simulink model "TCT_and_SUDOKU"  (R2025a)
settings: Solver=VariableStepAuto  StartTime=0.0  StopTime=1  RelTol=1e-3
libraries: spsDiodeLib x162, spsPVArrayLib x162, spsControlledVoltageSourceLib x2, spsCurrentMeasurementLib x2, simulink x2, spsVoltageMeasurementLib x2, sps_lib x1
(part 1 of 2)
settings Model: Creator=waquarahmad  LastModifiedBy=waquarahmad

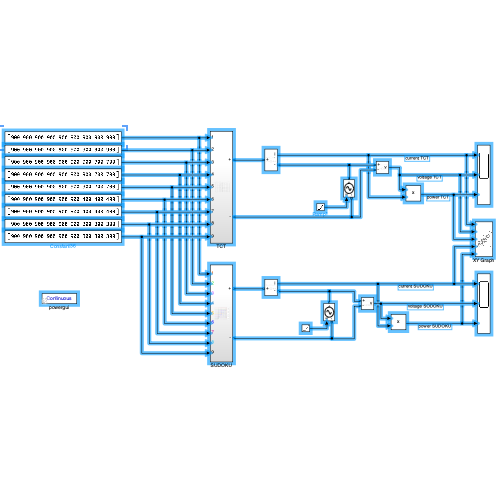
[thumbnail: Simulink's stored preview of the top-level diagram]
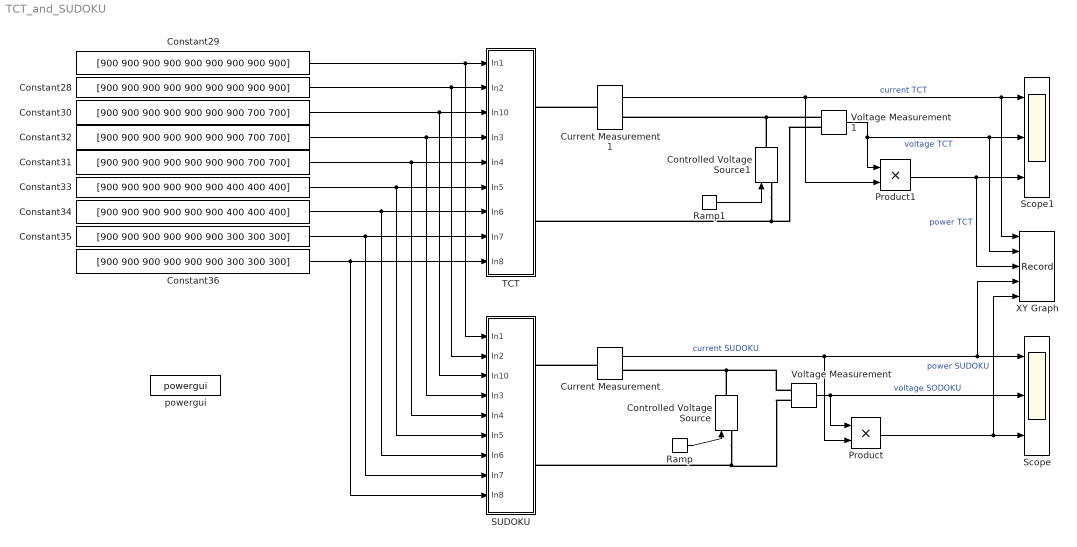
== system TCT_and_SUDOKU ==
  Constant28 : Constant  Value=[900 900 900 900 900 900 900 900 900]
  Constant29 : Constant  Value=[900 900 900 900 900 900 900 900 900]
  Constant30 : Constant  Value=[900 900 900 900 900 900 900 700 700]
  Constant31 : Constant  Value=[900 900 900 900 900 900 900 700 700]
  Constant32 : Constant  Value=[900 900 900 900 900 900 900 700 700]
  Constant33 : Constant  Value=[900 900 900 900 900 900 400 400 400]
  Constant34 : Constant  Value=[900 900 900 900 900 900 400 400 400]
  Constant35 : Constant  Value=[900 900 900 900 900 900 300 300 300]
  Constant36 : Constant  Value=[900 900 900 900 900 900 300 300 300]
  Controlled Voltage Source : spsControlledVoltageSourceLib/Controlled Voltage Source  Initialize=on  Source_Type=AC  Amplitude=0  Phase=0  Frequency=0  Measurements=None
  Controlled Voltage Source1 : spsControlledVoltageSourceLib/Controlled Voltage Source  Initialize=on  Source_Type=AC  Amplitude=0  Phase=0  Frequency=0  Measurements=None
  Current Measurement : spsCurrentMeasurementLib/Current Measurement  PhasorSimulation=off  OutputType=Complex  PSBequivalent=0
  Current Measurement1 : spsCurrentMeasurementLib/Current Measurement  PhasorSimulation=off  OutputType=Complex  PSBequivalent=0
  Product : Product
  Product1 : Product
  Ramp : simulink/Sources/Ramp  slope=22*9  start=0  InitialOutput=0
  Ramp1 : simulink/Sources/Ramp  slope=22*9  start=0  InitialOutput=0
  SUDOKU : Subsystem
  Scope : Scope  NumInputPorts=3
      settings: ActiveDisplayYMinimum=-11.703677982280553  ActiveDisplayYMaximum=43.6686902201964
  Scope1 : Scope  NumInputPorts=3
      settings: ActiveDisplayYMinimum=-1001.3880927326314  ActiveDisplayYMaximum=153.76114872783529
  TCT : Subsystem
  Voltage Measurement : spsVoltageMeasurementLib/Voltage Measurement  PhasorSimulation=off  OutputType=Complex  PSBequivalent=0
  Voltage Measurement1 : spsVoltageMeasurementLib/Voltage Measurement  PhasorSimulation=off  OutputType=Complex  PSBequivalent=0
  XY Graph : Record  NumPorts=5.0  FileSettingsInternal="{\"entries\":[{\"content\":{\"excelSettings\":{\"content\":{},\"type\":\"Streamout.ExcelSettings\"},\"parquetSettings\":{\"content\":{},\"type\":\"Streamout.ParquetSettings\"}},\"type\":\"Streamout.FileSettingStorage\",\"uuid\":\"\"}],\"packageUris\":[\"http:\\/\\/schema.mathworks.com\\/mf0\\/streamout_blocks\\/R2020a\"],\"version\":\"1.0\"}"  FrameSettings=[0, 0, 0, 0, 0]  Layout=[2 2]  SignalsInternal="{\"entries\":[{\"content\":{\"signals\":[{\"content\":{\"blockPath\":[],\"dimensions\":[1],\"domain\":\"\",\"lineColor\":\"#edb120\",\"lineWidth\":2,\"plots\":[ 2 ],\"port\":1,\"sid\":[\"\"],\"signalID\":1,\"signalName\":\"current TCT\"},\"type\":\"RecordBlkView.Signal\",\"uuid\":\"\"},{\"content\":{\"blockPath\":[],\"dimensions\":[1],\"domain\":\"\",\"lineColor\":\"#ff13a6\",\"lineWidth\":2,\"plots\":[ 1, 2 ],\"port\":2,\"sid\":[\"\"],\"signalID\":2,\"signalName\":\"voltage TCT\"},\"type\":\"RecordBlkView.Signal\",\"uuid\":\"\"},{\"content\":{\"blockPath\":[],\"dimensions\":[1],\"domain\":\"\",\"lineColor\":\"#fe330a\",\"lineWidth\":2,\"plots\":[ 1, 9 ],\"port\":3,\"sid\":[\"\"],\"signalID\":3,\"signalName\":\"power TCT\"},\"type\":\"RecordBlkView.Signal\",\"uuid\":\"\"},{\"content\":{\"blockPath\":[],\"dimensions\":[1],\"domain\":\"\",\"lineColor\":\"#22b573\",\"lineWidth\":2,\"plots\":[ 2 ],\"port\":4,\"sid\":[\"\"],\"signalID\":4,\"signalName\":\"current SUDOKU\"},\"type\":\"RecordBlkView.Signal\",\"uuid\":\"\"},{\"content\":{\"blockPath\":[],\"dimensions\":[1],\"domain\":\"\",\"lineColor\":\"#0072bd\",\"lineWidth\":2,\"plots\":[ 1, 10 ],\"port\":5,\"sid\":[\"\"],\"signalID\":5,\"signalName\":\"power SUDOKU\"},\"type\":\"RecordBlkView.Signal\",\"uuid\":\"\"}]},\"type\":\"RecordBlkView.InputSignals\",\"uuid\":\"\"}],\"packageUris\":[\"http:\\/\\/schema.mathworks.com\\/mf0\\/streamout_blocks\\/R2020a\"],\"version\":\"1.0\"}"  VisualizationBindings="{\"xyplotplugin\":{\"info\":[{\"series\":[{\"bindingParametersList\":[{\"parameter\":\"X-Axis\",\"signalID\":2,\"signalName\":\"voltage TCT\"},{\"parameter\":\"Y-Axis\",\"signalID\":5,\"signalName\":\"power SUDOKU\"},{\"parameter\":\"X-Axis\",\"signalID\":2,\"signalName\":\"voltage TCT\"},{\"parameter\":\"Y-Axis\",\"signalID\":5,\"signalName\":\"power SUDOKU\"}],\"seriesID\":0},{\"bindingParametersList\":[{\"parameter\":\"X-Axis\",\"signalID\":2,\"signalName\":\"voltage TCT\"},{\"parameter\":\"Y-Axis\",\"signalID\":3,\"signalName\":\"power TCT\"},{\"parameter\":\"X-Axis\",\"signalID\":2,\"signalName\":\"voltage TCT\"},{\"parameter\":\"Y-Axis\",\"signalID\":3,\"signalName\":\"power TCT\"}],\"seriesID\":1}],\"subplotID\":1},{\"series\":[{\"bindingParametersList\":[{\"parameter\":\"X-Axis\",\"signalID\":2,\"signalName\":\"voltage TCT\"},{\"parameter\":\"Y-Axis\",\"signalID\":1,\"signalName\":\"current TCT\"}],\"seriesID\":2},{\"bindingParametersList\":[{\"parameter\":\"X-Axis\",\"signalID\":2,\"signalName\":\"voltage TCT\"},{\"parameter\":\"Y-Axis\",\"signalID\":4,\"signalName\":\"current SUDOKU\"}],\"seriesID\":3}],\"subplotID\":2}]}}"  CompatibilityTag=XY
  powergui : sps_lib/powergui  Priority=1  SimulationMode=Continuous  SampleTime=1e-5  frequency=60  Iterations=50  frequencyindice=0  Pbase=100e6  ErrMax=1e-4  UnitsV=kV  UnitsW=MW  buscounter=0  FunctionMessages=off  echomessages=off  EnableUseOfTLC=off  CurrentSourceSwitches=off  DisableSnubberDevices=off  DisableRonSwitches=off  DisableVfSwitches=off  DisplayEquations=off  AutomaticDiscreteSolvers=off  SolverType=Tustin/Backward Euler (TBE)  Interpol=off  ExternalGateDelay=off  methode=off  Ts=100  x0status=blocks  SPID=on  SwTol=0  HookPort=off  NonlinearTolerance=1e-4  nMaxIteration=100  ContinueOnMaxIteration=off  RestoreLinks=warning  ResistiveCurrentMeasurement=off  Frange=[0:2:500]  Ylog=off  Xlog=on  ShowGrid=off  save=off  variable=ZData  structure=0  ZoomFFT=off  StartTime=0.0  cycles=1  DisplayStyle=1  fundamental=60  FreqAxis=off  MaxFrequency=1000  frequencyindicesteady=1  RmsSteady=1  display=off
  wires:
  Product/1 -> XY Graph/5, Scope/3  "power SUDOKU"
  Ramp/1 -> Controlled Voltage Source/1
  Voltage Measurement/1 -> Product/1, Scope/2  "voltage SODOKU"
  Current Measurement/1 -> Scope/1, XY Graph/4, Product/2  "current SUDOKU"
  Constant34/1 -> SUDOKU/7(In6), TCT/7(In6)
  Constant32/1 -> SUDOKU/4(In3), TCT/4(In3)
  Constant36/1 -> SUDOKU/9(In8), TCT/9(In8)
  Constant28/1 -> SUDOKU/2(In2), TCT/2(In2)
  Constant35/1 -> SUDOKU/8(In7), TCT/8(In7)
  Ramp1/1 -> Controlled Voltage Source1/1
  Product1/1 -> XY Graph/3, Scope1/3  "power TCT"
  Constant29/1 -> SUDOKU/1(In1), TCT/1(In1)
  Constant31/1 -> SUDOKU/5(In4), TCT/5(In4)
  Voltage Measurement1/1 -> Product1/1, XY Graph/2, Scope1/2  "voltage TCT"
  Constant33/1 -> SUDOKU/6(In5), TCT/6(In5)
  Constant30/1 -> SUDOKU/3(In10), TCT/3(In10)
  Current Measurement1/1 -> Product1/2, XY Graph/1, Scope1/1  "current TCT"
  connections:
  Controlled Voltage Source/RConn1 -- Voltage Measurement/LConn1 -- Current Measurement/RConn1
  Voltage Measurement/LConn2 -- Controlled Voltage Source/LConn1 -- SUDOKU/RConn2
  Current Measurement/LConn1 -- SUDOKU/RConn1
  Controlled Voltage Source1/RConn1 -- Voltage Measurement1/LConn1 -- Current Measurement1/RConn1
  Voltage Measurement1/LConn2 -- TCT/RConn2 -- Controlled Voltage Source1/LConn1
  Current Measurement1/LConn1 -- TCT/RConn1

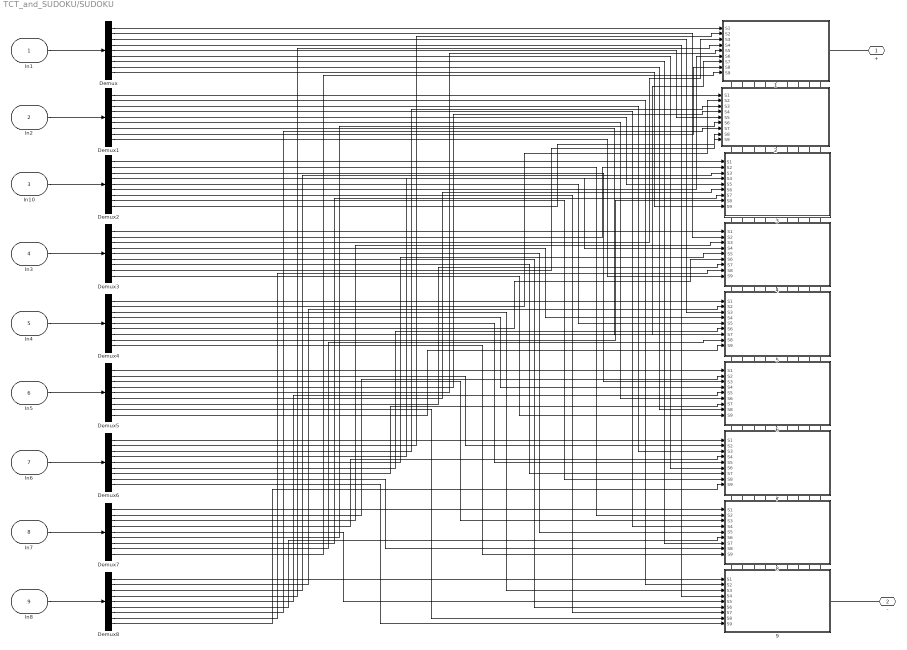
== system TCT_and_SUDOKU/SUDOKU ==
  In1 : Inport
  In2 : Inport  Port=2
  In10 : Inport  Port=3
  In3 : Inport  Port=4
  In4 : Inport  Port=5
  In5 : Inport  Port=6
  In6 : Inport  Port=7
  In7 : Inport  Port=8
  In8 : Inport  Port=9
  1 : Subsystem
      settings: PortSchema="{\"entries\":[{\"content\":{\"sides\":[{\"content\":{\"connectorIds\":[\"In1\",\"In2\",\"In3\",\"In4\",\"In5\",\"In6\",\"In7\",\"In8\",\"In9\"]},\"type\":\"ConnectorPlacement.EquallySpacedRectSide\",\"uuid\":\"947c48e2-5623-469f-a5b5-f7fc9c96f3a0\"},{\"content\":{\"connectorIds\":[\"RConn1\"],\"side\":\"RIGHT\"},\"type\":\"ConnectorPlacement.EquallySpacedRectSide\",\"uuid\":\"a3fb3b29-0daa-4d0d-9d6d-8bc671be3af7\"},{\"content\":{\"side\":\"TOP\"},\"type\":\"ConnectorPlacement.EquallySpacedRectSide\",\"uuid\":\"d19fbb75-5505-4b73-a602-811c913b3a41\"},{\"content\":{\"connectorIds\":[\"RConn2\",\"RConn3\",\"RConn4\",\"RConn5\",\"RConn6\",\"RConn7\",\"RConn8\",\"RConn9\",\"RConn10\"],\"side\":\"BOTTOM\"},\"type\":\"ConnectorPlacement.EquallySpacedRectSide\",\"uuid\":\"978d761e-6adc-4ec8-8d47-d13e72af1dc0\"}]},\"type\":\"ConnectorPlacement.EquallySpacedConnector\",\"uuid\":\"4602dd69-8142-41e9-90b3-db6b24cf4d7a\"}],\"packageUris\":[\"http://schema.mathworks.com/mf0/Connector/R2020b\"],\"version\":\"1.0\"}"
  2 : Subsystem
      settings: PortSchema="{\"entries\":[{\"content\":{\"sides\":[{\"content\":{\"connectorIds\":[\"LConn1\",\"LConn2\",\"LConn3\",\"LConn4\",\"LConn5\",\"LConn6\",\"LConn7\",\"LConn8\",\"LConn9\"]},\"type\":\"ConnectorPlacement.EquallySpacedRectSide\",\"uuid\":\"a8afa343-d22f-48fe-a0b1-87abb85ad042\"},{\"content\":{\"connectorIds\":[\"RConn1\",\"RConn2\",\"RConn3\",\"RConn4\",\"RConn5\",\"RConn6\",\"RConn7\",\"RConn8\",\"RConn9\"],\"side\":\"RIGHT\"},\"type\":\"ConnectorPlacement.EquallySpacedRectSide\",\"uuid\":\"78b1e069-c992-4391-bbef-a9be779e1125\"},{\"content\":{\"connectorIds\":[\"In1\",\"In2\",\"In3\",\"In4\",\"In5\",\"In6\",\"In7\",\"In8\",\"In9\"],\"side\":\"TOP\"},\"type\":\"ConnectorPlacement.EquallySpacedRectSide\",\"uuid\":\"2312311a-78a4-4c80-802a-cd67b6e84b86\"}]},\"type\":\"ConnectorPlacement.EquallySpacedConnector\",\"uuid\":\"0b9d0645-d0b0-4ada-9e60-692c847bbde6\"}],\"packageUris\":[\"http://schema.mathworks.com/mf0/Connector/R2020b\"],\"version\":\"1.0\"}"
  3 : Subsystem
      settings: PortSchema="{\"entries\":[{\"content\":{\"sides\":[{\"content\":{\"connectorIds\":[\"LConn1\",\"LConn2\",\"LConn3\",\"LConn4\",\"LConn5\",\"LConn6\",\"LConn7\",\"LConn8\",\"LConn9\"]},\"type\":\"ConnectorPlacement.EquallySpacedRectSide\",\"uuid\":\"a8afa343-d22f-48fe-a0b1-87abb85ad042\"},{\"content\":{\"connectorIds\":[\"RConn1\",\"RConn2\",\"RConn3\",\"RConn4\",\"RConn5\",\"RConn6\",\"RConn7\",\"RConn8\",\"RConn9\"],\"side\":\"RIGHT\"},\"type\":\"ConnectorPlacement.EquallySpacedRectSide\",\"uuid\":\"78b1e069-c992-4391-bbef-a9be779e1125\"},{\"content\":{\"connectorIds\":[\"In1\",\"In2\",\"In3\",\"In4\",\"In5\",\"In6\",\"In7\",\"In8\",\"In9\"],\"side\":\"TOP\"},\"type\":\"ConnectorPlacement.EquallySpacedRectSide\",\"uuid\":\"2312311a-78a4-4c80-802a-cd67b6e84b86\"}]},\"type\":\"ConnectorPlacement.EquallySpacedConnector\",\"uuid\":\"0b9d0645-d0b0-4ada-9e60-692c847bbde6\"}],\"packageUris\":[\"http://schema.mathworks.com/mf0/Connector/R2020b\"],\"version\":\"1.0\"}"
  4 : Subsystem
      settings: PortSchema="{\"entries\":[{\"content\":{\"sides\":[{\"content\":{\"connectorIds\":[\"LConn1\",\"LConn2\",\"LConn3\",\"LConn4\",\"LConn5\",\"LConn6\",\"LConn7\",\"LConn8\",\"LConn9\"]},\"type\":\"ConnectorPlacement.EquallySpacedRectSide\",\"uuid\":\"a8afa343-d22f-48fe-a0b1-87abb85ad042\"},{\"content\":{\"connectorIds\":[\"RConn1\",\"RConn2\",\"RConn3\",\"RConn4\",\"RConn5\",\"RConn6\",\"RConn7\",\"RConn8\",\"RConn9\"],\"side\":\"RIGHT\"},\"type\":\"ConnectorPlacement.EquallySpacedRectSide\",\"uuid\":\"78b1e069-c992-4391-bbef-a9be779e1125\"},{\"content\":{\"connectorIds\":[\"In1\",\"In2\",\"In3\",\"In4\",\"In5\",\"In6\",\"In7\",\"In8\",\"In9\"],\"side\":\"TOP\"},\"type\":\"ConnectorPlacement.EquallySpacedRectSide\",\"uuid\":\"2312311a-78a4-4c80-802a-cd67b6e84b86\"}]},\"type\":\"ConnectorPlacement.EquallySpacedConnector\",\"uuid\":\"0b9d0645-d0b0-4ada-9e60-692c847bbde6\"}],\"packageUris\":[\"http://schema.mathworks.com/mf0/Connector/R2020b\"],\"version\":\"1.0\"}"
  5 : Subsystem
      settings: PortSchema="{\"entries\":[{\"content\":{\"sides\":[{\"content\":{\"connectorIds\":[\"LConn1\",\"LConn2\",\"LConn3\",\"LConn4\",\"LConn5\",\"LConn6\",\"LConn7\",\"LConn8\",\"LConn9\"]},\"type\":\"ConnectorPlacement.EquallySpacedRectSide\",\"uuid\":\"a8afa343-d22f-48fe-a0b1-87abb85ad042\"},{\"content\":{\"connectorIds\":[\"RConn1\",\"RConn2\",\"RConn3\",\"RConn4\",\"RConn5\",\"RConn6\",\"RConn7\",\"RConn8\",\"RConn9\"],\"side\":\"RIGHT\"},\"type\":\"ConnectorPlacement.EquallySpacedRectSide\",\"uuid\":\"78b1e069-c992-4391-bbef-a9be779e1125\"},{\"content\":{\"connectorIds\":[\"In1\",\"In2\",\"In3\",\"In4\",\"In5\",\"In6\",\"In7\",\"In8\",\"In9\"],\"side\":\"TOP\"},\"type\":\"ConnectorPlacement.EquallySpacedRectSide\",\"uuid\":\"2312311a-78a4-4c80-802a-cd67b6e84b86\"}]},\"type\":\"ConnectorPlacement.EquallySpacedConnector\",\"uuid\":\"0b9d0645-d0b0-4ada-9e60-692c847bbde6\"}],\"packageUris\":[\"http://schema.mathworks.com/mf0/Connector/R2020b\"],\"version\":\"1.0\"}"
  6 : Subsystem
      settings: PortSchema="{\"entries\":[{\"content\":{\"sides\":[{\"content\":{\"connectorIds\":[\"LConn1\",\"LConn2\",\"LConn3\",\"LConn4\",\"LConn5\",\"LConn6\",\"LConn7\",\"LConn8\",\"LConn9\"]},\"type\":\"ConnectorPlacement.EquallySpacedRectSide\",\"uuid\":\"a8afa343-d22f-48fe-a0b1-87abb85ad042\"},{\"content\":{\"connectorIds\":[\"RConn1\",\"RConn2\",\"RConn3\",\"RConn4\",\"RConn5\",\"RConn6\",\"RConn7\",\"RConn8\",\"RConn9\"],\"side\":\"RIGHT\"},\"type\":\"ConnectorPlacement.EquallySpacedRectSide\",\"uuid\":\"78b1e069-c992-4391-bbef-a9be779e1125\"},{\"content\":{\"connectorIds\":[\"In1\",\"In2\",\"In3\",\"In4\",\"In5\",\"In6\",\"In7\",\"In8\",\"In9\"],\"side\":\"TOP\"},\"type\":\"ConnectorPlacement.EquallySpacedRectSide\",\"uuid\":\"2312311a-78a4-4c80-802a-cd67b6e84b86\"}]},\"type\":\"ConnectorPlacement.EquallySpacedConnector\",\"uuid\":\"0b9d0645-d0b0-4ada-9e60-692c847bbde6\"}],\"packageUris\":[\"http://schema.mathworks.com/mf0/Connector/R2020b\"],\"version\":\"1.0\"}"
  7 : Subsystem
      settings: PortSchema="{\"entries\":[{\"content\":{\"sides\":[{\"content\":{\"connectorIds\":[\"LConn1\",\"LConn2\",\"LConn3\",\"LConn4\",\"LConn5\",\"LConn6\",\"LConn7\",\"LConn8\",\"LConn9\"]},\"type\":\"ConnectorPlacement.EquallySpacedRectSide\",\"uuid\":\"a8afa343-d22f-48fe-a0b1-87abb85ad042\"},{\"content\":{\"connectorIds\":[\"RConn1\",\"RConn2\",\"RConn3\",\"RConn4\",\"RConn5\",\"RConn6\",\"RConn7\",\"RConn8\",\"RConn9\"],\"side\":\"RIGHT\"},\"type\":\"ConnectorPlacement.EquallySpacedRectSide\",\"uuid\":\"78b1e069-c992-4391-bbef-a9be779e1125\"},{\"content\":{\"connectorIds\":[\"In1\",\"In2\",\"In3\",\"In4\",\"In5\",\"In6\",\"In7\",\"In8\",\"In9\"],\"side\":\"TOP\"},\"type\":\"ConnectorPlacement.EquallySpacedRectSide\",\"uuid\":\"2312311a-78a4-4c80-802a-cd67b6e84b86\"}]},\"type\":\"ConnectorPlacement.EquallySpacedConnector\",\"uuid\":\"0b9d0645-d0b0-4ada-9e60-692c847bbde6\"}],\"packageUris\":[\"http://schema.mathworks.com/mf0/Connector/R2020b\"],\"version\":\"1.0\"}"
  8 : Subsystem
      settings: PortSchema="{\"entries\":[{\"content\":{\"sides\":[{\"content\":{\"connectorIds\":[\"LConn1\",\"LConn2\",\"LConn3\",\"LConn4\",\"LConn5\",\"LConn6\",\"LConn7\",\"LConn8\",\"LConn9\"]},\"type\":\"ConnectorPlacement.EquallySpacedRectSide\",\"uuid\":\"a8afa343-d22f-48fe-a0b1-87abb85ad042\"},{\"content\":{\"connectorIds\":[\"RConn1\",\"RConn2\",\"RConn3\",\"RConn4\",\"RConn5\",\"RConn6\",\"RConn7\",\"RConn8\",\"RConn9\"],\"side\":\"RIGHT\"},\"type\":\"ConnectorPlacement.EquallySpacedRectSide\",\"uuid\":\"78b1e069-c992-4391-bbef-a9be779e1125\"},{\"content\":{\"connectorIds\":[\"In1\",\"In2\",\"In3\",\"In4\",\"In5\",\"In6\",\"In7\",\"In8\",\"In9\"],\"side\":\"TOP\"},\"type\":\"ConnectorPlacement.EquallySpacedRectSide\",\"uuid\":\"2312311a-78a4-4c80-802a-cd67b6e84b86\"}]},\"type\":\"ConnectorPlacement.EquallySpacedConnector\",\"uuid\":\"0b9d0645-d0b0-4ada-9e60-692c847bbde6\"}],\"packageUris\":[\"http://schema.mathworks.com/mf0/Connector/R2020b\"],\"version\":\"1.0\"}"
  9 : Subsystem
      settings: PortSchema="{\"entries\":[{\"content\":{\"sides\":[{\"content\":{},\"type\":\"ConnectorPlacement.EquallySpacedRectSide\",\"uuid\":\"e7f2cbc5-ad1c-43d4-bf0d-1483c7381513\"},{\"content\":{\"connectorIds\":[\"RConn1\",\"RConn2\",\"RConn3\",\"RConn4\",\"RConn5\",\"RConn6\",\"RConn7\",\"RConn8\",\"RConn9\"],\"side\":\"RIGHT\"},\"type\":\"ConnectorPlacement.EquallySpacedRectSide\",\"uuid\":\"5a9a4e7c-59bb-4c28-84ef-2febbfad019a\"},{\"content\":{\"connectorIds\":[\"In1\",\"In2\",\"In3\",\"In4\",\"In5\",\"In6\",\"In7\",\"In8\",\"In9\"],\"side\":\"TOP\"},\"type\":\"ConnectorPlacement.EquallySpacedRectSide\",\"uuid\":\"b37d546a-1546-4b2a-9237-35eddc952232\"},{\"content\":{\"connectorIds\":[\"RConn10\"],\"side\":\"BOTTOM\"},\"type\":\"ConnectorPlacement.EquallySpacedRectSide\",\"uuid\":\"f9c0eeef-80c0-4604-a732-477139749fca\"}]},\"type\":\"ConnectorPlacement.EquallySpacedConnector\",\"uuid\":\"79c82ad3-5495-4616-9c09-f0403446a694\"}],\"packageUris\":[\"http://schema.mathworks.com/mf0/Connector/R2020b\"],\"version\":\"1.0\"}"
  Demux{,1..8} (9 alike) : Demux  Outputs=9
  + : PMIOPort  Side=Right
  - : PMIOPort  Port=2  Side=Right
  wires:
  Demux/1 -> 1/1(S1)
  Demux/2 -> 4/8(S2)
  Demux/3 -> 5/7(S3)
  Demux/4 -> 9/6(S4)
  Demux/5 -> 2/5(S5)
  Demux/6 -> 7/4(S6)
  Demux/7 -> 8/3(S7)
  Demux/8 -> 6/2(S8)
  Demux/9 -> 3/1(S9)
  Demux1/1 -> 2/9(S1)
  Demux1/2 -> 9/8(S2)
  Demux1/3 -> 7/7(S3)
  Demux1/4 -> 8/6(S4)
  Demux1/5 -> 3/5(S5)
  Demux1/6 -> 6/4(S6)
  Demux1/7 -> 5/3(S7)
  Demux1/8 -> 1/8(S8)
  Demux1/9 -> 4/1(S9)
  Demux2/1 -> 3/9(S1)
  Demux2/2 -> 8/8(S2)
  Demux2/3 -> 6/7(S3)
  Demux2/4 -> 4/6(S4)
  Demux2/5 -> 5/5(S5)
  Demux2/6 -> 1/6(S6)
  Demux2/7 -> 9/3(S7)
  Demux2/8 -> 7/2(S8)
  Demux2/9 -> 2/1(S9)
  Demux3/1 -> 4/9(S1)
  Demux3/2 -> 3/8(S2)
  Demux3/3 -> 1/3(S3)
  Demux3/4 -> 5/6(S4)
  Demux3/5 -> 8/5(S5)
  Demux3/6 -> 9/4(S6)
  Demux3/7 -> 7/3(S7)
  Demux3/8 -> 2/2(S8)
  Demux3/9 -> 6/1(S9)
  Demux4/1 -> 5/9(S1)
  Demux4/2 -> 2/8(S2)
  Demux4/3 -> 9/7(S3)
  Demux4/4 -> 6/6(S4)
  Demux4/5 -> 7/5(S5)
  Demux4/6 -> 4/4(S6)
  Demux4/7 -> 1/7(S7)
  Demux4/8 -> 3/2(S8)
  Demux4/9 -> 8/1(S9)
  Demux5/1 -> 6/9(S1)
  Demux5/2 -> 7/8(S2)
  Demux5/3 -> 8/7(S3)
  Demux5/4 -> 2/6(S4)
  Demux5/5 -> 1/5(S5)
  Demux5/6 -> 3/4(S6)
  Demux5/7 -> 4/3(S7)
  Demux5/8 -> 9/2(S8)
  Demux5/9 -> 5/1(S9)
  Demux6/1 -> 7/9(S1)
  Demux6/2 -> 1/2(S2)
  Demux6/3 -> 2/7(S3)
  Demux6/4 -> 3/6(S4)
  Demux6/5 -> 4/5(S5)
  Demux6/6 -> 5/4(S6)
  Demux6/7 -> 6/3(S7)
  Demux6/8 -> 8/2(S8)
  Demux6/9 -> 9/1(S9)
  Demux7/1 -> 8/9(S1)
  Demux7/2 -> 6/8(S2)
  Demux7/3 -> 4/7(S3)
  Demux7/4 -> 7/6(S4)
  Demux7/5 -> 9/5(S5)
  Demux7/6 -> 2/4(S6)
  Demux7/7 -> 3/3(S7)
  Demux7/8 -> 5/2(S8)
  Demux7/9 -> 1/9(S9)
  Demux8/1 -> 9/9(S1)
  Demux8/2 -> 5/8(S2)
  Demux8/3 -> 3/7(S3)
  Demux8/4 -> 1/4(S4)
  Demux8/5 -> 6/5(S5)
  Demux8/6 -> 8/4(S6)
  Demux8/7 -> 2/3(S7)
  Demux8/8 -> 4/2(S8)
  Demux8/9 -> 7/1(S9)
  In1/1 -> Demux/1
  In2/1 -> Demux1/1
  In10/1 -> Demux2/1
  In3/1 -> Demux3/1
  In4/1 -> Demux4/1
  In5/1 -> Demux5/1
  In6/1 -> Demux6/1
  In7/1 -> Demux7/1
  In8/1 -> Demux8/1
  connections:
  +/RConn1 -- 1/RConn1
  2/RConn1 -- 1/RConn2
  2/RConn2 -- 1/RConn3
  2/RConn3 -- 1/RConn4
  2/RConn4 -- 1/RConn5
  2/RConn5 -- 1/RConn6
  2/RConn6 -- 1/RConn7
  2/RConn7 -- 1/RConn8
  2/RConn8 -- 1/RConn9
  1/RConn10 -- 2/RConn9
  3/RConn1 -- 2/LConn1
  3/RConn2 -- 2/LConn2
  2/LConn3 -- 3/RConn3
  2/LConn4 -- 3/RConn4
  2/LConn5 -- 3/RConn5
  2/LConn6 -- 3/RConn6
  2/LConn7 -- 3/RConn7
  2/LConn8 -- 3/RConn8
  2/LConn9 -- 3/RConn9
  4/RConn1 -- 3/LConn1
  4/RConn2 -- 3/LConn2
  3/LConn3 -- 4/RConn3
  4/RConn4 -- 3/LConn4
  3/LConn5 -- 4/RConn5
  3/LConn6 -- 4/RConn6
  3/LConn7 -- 4/RConn7
  3/LConn8 -- 4/RConn8
  3/LConn9 -- 4/RConn9
  5/RConn1 -- 4/LConn1
  5/RConn2 -- 4/LConn2
  5/RConn3 -- 4/LConn3
  5/RConn4 -- 4/LConn4
  5/RConn5 -- 4/LConn5
  5/RConn6 -- 4/LConn6
  5/RConn7 -- 4/LConn7
  5/RConn8 -- 4/LConn8
  5/RConn9 -- 4/LConn9
  6/RConn1 -- 5/LConn1
  6/RConn2 -- 5/LConn2
  6/RConn3 -- 5/LConn3
  6/RConn4 -- 5/LConn4
  6/RConn5 -- 5/LConn5
  6/RConn6 -- 5/LConn6
  6/RConn7 -- 5/LConn7
  6/RConn8 -- 5/LConn8
  6/RConn9 -- 5/LConn9
  7/RConn1 -- 6/LConn1
  7/RConn2 -- 6/LConn2
  6/LConn3 -- 7/RConn3
  7/RConn4 -- 6/LConn4
  7/RConn5 -- 6/LConn5
  7/RConn6 -- 6/LConn6
  7/RConn7 -- 6/LConn7
  7/RConn8 -- 6/LConn8
  7/RConn9 -- 6/LConn9
  7/LConn1 -- 8/RConn1
  8/RConn2 -- 7/LConn2
  8/RConn3 -- 7/LConn3
  8/RConn4 -- 7/LConn4
  8/RConn5 -- 7/LConn5
  8/RConn6 -- 7/LConn6
  8/RConn7 -- 7/LConn7
  8/RConn8 -- 7/LConn8
  8/RConn9 -- 7/LConn9
  9/RConn1 -- 8/LConn1
  9/RConn2 -- 8/LConn2
  9/RConn3 -- 8/LConn3
  9/RConn4 -- 8/LConn4
  9/RConn5 -- 8/LConn5
  9/RConn6 -- 8/LConn6
  9/RConn7 -- 8/LConn7
  9/RConn8 -- 8/LConn8
  9/RConn9 -- 8/LConn9
  -/RConn1 -- 9/RConn10

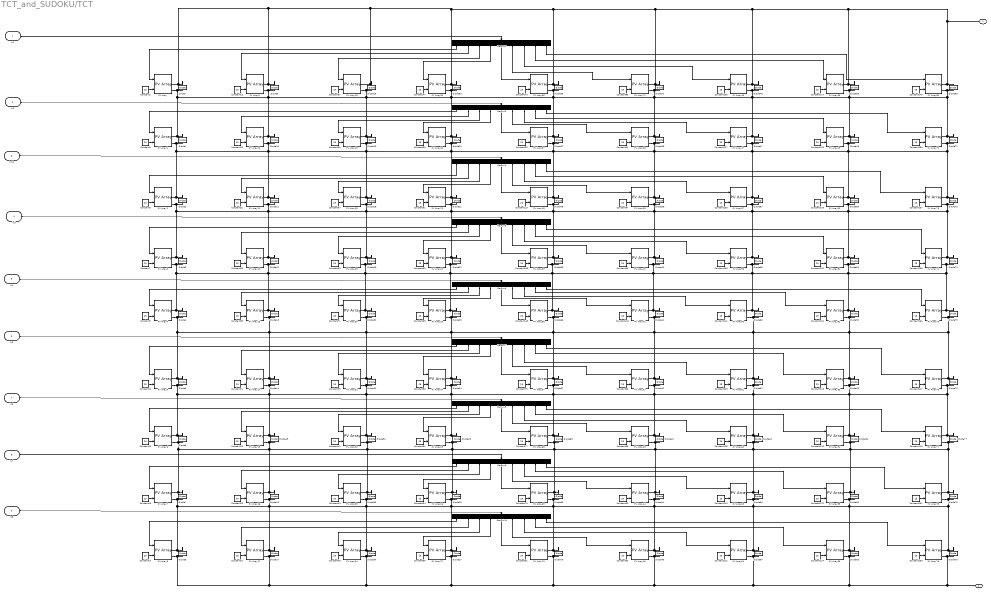
== system TCT_and_SUDOKU/TCT ==
  In1 : Inport
  In2 : Inport  Port=2
  In10 : Inport  Port=3
  In3 : Inport  Port=4
  In4 : Inport  Port=5
  In5 : Inport  Port=6
  In6 : Inport  Port=7
  In7 : Inport  Port=8
  In8 : Inport  Port=9
  Constant{1,3,5,7,9,11,13,15,17,19,21,23,25,27,29,31,33,35,37,39,41,43,45,47,50,52,54,56,58..59,61,63,65,67,69,71,73,75,77,79,81,83,86,88,90,92,94..95,97,99,101,103,105,108,110,112,114,117..118,120,122,124,126..127,130,132,134,136,138..139,141,143,145,147,149,151,153,155,157,159,161} (81 alike) : Constant  Value=25
  Demux{2..10} (9 alike) : Demux  Outputs=9
  Diode{,1..80} (81 alike) : spsDiodeLib/Diode  Ron=0.001  Lon=0  Vf=0.8  IC=0  UseSnubber=0  Rs=500  Cs=250e-9  Measurements=off
  PV Array{,1..80} (81 alike) : spsPVArrayLib/PV Array  Npar=1  Nser=1  PlotType=array @ 1000 W/m2 & specified temperatures  S_vec="[ 1000  500  100 ]"  Temp_C_vec="[ 45 25  ]"  ModuleName=User-defined  PlotWhenSelected=off  Pm=79.2  Ncell=60  Voc=22  Isc=4.7  Vm=18  Im=4.4  beta_Voc_pc=-0.36099  alpha_Isc_pc=0.102  beta_Voc=-0.079418  alpha_Isc=0.004794  IL=4.7103  I0=1.7336e-10  nI=0.59447  Rsh=255.4401  Rs=0.29081  RobustModel=off  RobustCellTemperature=313.3991  BAL=on  Tc=1e-6  Tfilter=5e-5
  + : PMIOPort  Side=Right
  - : PMIOPort  Port=2  Side=Right
  wires:
  Constant134/1 -> PV Array52/2
  Constant151/1 -> PV Array78/2
  Constant112/1 -> PV Array64/2
  Constant145/1 -> PV Array80/2
  Constant161/1 -> PV Array75/2
  Constant138/1 -> PV Array58/2
  Constant153/1 -> PV Array79/2
  Constant159/1 -> PV Array74/2
  Constant13/1 -> PV Array6/2
  Constant103/1 -> PV Array46/2
  Constant77/1 -> PV Array68/2
  Constant157/1 -> PV Array73/2
  Constant5/1 -> PV Array2/2
  Constant105/1 -> PV Array61/2
  Constant124/1 -> PV Array56/2
  Constant130/1 -> PV Array50/2
  Constant141/1 -> PV Array60/2
  Constant126/1 -> PV Array49/2
  Constant120/1 -> PV Array54/2
  Constant149/1 -> PV Array77/2
  Constant17/1 -> PV Array8/2
  Constant92/1 -> PV Array45/2
  Constant86/1 -> PV Array42/2
  Constant117/1 -> PV Array48/2
  Constant95/1 -> PV Array37/2
  Constant108/1 -> PV Array62/2
  Constant155/1 -> PV Array72/2
  Constant122/1 -> PV Array55/2
  Constant35/1 -> PV Array13/2
  Constant139/1 -> PV Array59/2
  Constant65/1 -> PV Array23/2
  Constant58/1 -> PV Array20/2
  Constant52/1 -> PV Array25/2
  Constant61/1 -> PV Array21/2
  Constant97/1 -> PV Array39/2
  Constant71/1 -> PV Array30/2
  Constant3/1 -> PV Array1/2
  Constant7/1 -> PV Array3/2
  Constant25/1 -> PV Array16/2
  Constant63/1 -> PV Array22/2
  Constant43/1 -> PV Array33/2
  Constant9/1 -> PV Array4/2
  Constant29/1 -> PV Array10/2
  Constant88/1 -> PV Array43/2
  Constant99/1 -> PV Array40/2
  Constant83/1 -> PV Array71/2
  Constant127/1 -> PV Array47/2
  Constant59/1 -> PV Array19/2
  Constant1/1 -> PV Array/2
  Constant147/1 -> PV Array76/2
  Constant31/1 -> PV Array11/2
  Constant90/1 -> PV Array44/2
  Constant11/1 -> PV Array5/2
  Constant21/1 -> PV Array14/2
  Constant67/1 -> PV Array28/2
  Constant114/1 -> PV Array65/2
  Constant27/1 -> PV Array17/2
  Constant132/1 -> PV Array51/2
  Constant45/1 -> PV Array34/2
  Constant79/1 -> PV Array69/2
  Constant69/1 -> PV Array29/2
  Constant50/1 -> PV Array24/2
  Constant56/1 -> PV Array27/2
  Constant47/1 -> PV Array35/2
  Constant37/1 -> PV Array18/2
  Constant39/1 -> PV Array31/2
  Constant33/1 -> PV Array12/2
  Constant73/1 -> PV Array36/2
  Constant23/1 -> PV Array15/2
  Constant94/1 -> PV Array38/2
  Constant118/1 -> PV Array53/2
  Constant19/1 -> PV Array9/2
  Constant136/1 -> PV Array57/2
  Constant143/1 -> PV Array66/2
  Constant75/1 -> PV Array67/2
  Constant110/1 -> PV Array63/2
  Constant101/1 -> PV Array41/2
  Constant41/1 -> PV Array32/2
  Constant54/1 -> PV Array26/2
  Constant81/1 -> PV Array70/2
  Constant15/1 -> PV Array7/2
  In1/1 -> Demux2/1
  Demux2/1 -> PV Array/1
  Demux2/2 -> PV Array9/1
  Demux3/1 -> PV Array1/1
  Demux3/2 -> PV Array10/1
  Demux3/3 -> PV Array19/1
  Demux3/4 -> PV Array20/1
  Demux3/5 -> PV Array37/1
  Demux3/6 -> PV Array38/1
  Demux3/7 -> PV Array47/1
  Demux2/3 -> PV Array18/1
  Demux2/4 -> PV Array35/1
  Demux2/5 -> PV Array36/1
  Demux2/6 -> PV Array71/1
  Demux2/7 -> PV Array46/1
  Demux2/8 -> PV Array65/1
  Demux2/9 -> PV Array80/1
  Demux3/9 -> PV Array72/1
  Demux3/8 -> PV Array49/1
  Demux4/1 -> PV Array2/1
  Demux4/2 -> PV Array11/1
  Demux4/3 -> PV Array28/1
  Demux4/4 -> PV Array21/1
  Demux4/5 -> PV Array48/1
  Demux4/6 -> PV Array39/1
  Demux4/7 -> PV Array57/1
  Demux4/8 -> PV Array50/1
  Demux4/9 -> PV Array73/1
  Demux5/1 -> PV Array3/1
  Demux5/2 -> PV Array12/1
  Demux5/3 -> PV Array29/1
  Demux5/4 -> PV Array22/1
  Demux5/5 -> PV Array59/1
  Demux5/6 -> PV Array40/1
  Demux5/7 -> PV Array58/1
  Demux5/8 -> PV Array51/1
  Demux5/9 -> PV Array74/1
  Demux6/1 -> PV Array4/1
  Demux6/2 -> PV Array13/1
  Demux6/3 -> PV Array30/1
  Demux6/4 -> PV Array23/1
  Demux6/5 -> PV Array66/1
  Demux6/6 -> PV Array41/1
  Demux6/7 -> PV Array60/1
  Demux6/8 -> PV Array52/1
  Demux6/9 -> PV Array75/1
  Demux7/1 -> PV Array5/1
  Demux7/2 -> PV Array14/1
  Demux7/3 -> PV Array31/1
  Demux7/4 -> PV Array24/1
  Demux7/5 -> PV Array67/1
  Demux7/6 -> PV Array42/1
  Demux7/7 -> PV Array61/1
  Demux7/8 -> PV Array53/1
  Demux7/9 -> PV Array76/1
  Demux8/1 -> PV Array6/1
  Demux8/2 -> PV Array15/1
  Demux8/3 -> PV Array32/1
  Demux8/4 -> PV Array25/1
  Demux8/5 -> PV Array68/1
  Demux8/6 -> PV Array43/1
  Demux8/7 -> PV Array62/1
  Demux8/8 -> PV Array54/1
  Demux8/9 -> PV Array77/1
  Demux9/1 -> PV Array7/1
  Demux9/2 -> PV Array16/1
  Demux9/3 -> PV Array33/1
  Demux9/4 -> PV Array26/1
  Demux9/5 -> PV Array69/1
  Demux9/6 -> PV Array44/1
  Demux9/7 -> PV Array63/1
  Demux9/8 -> PV Array55/1
  Demux9/9 -> PV Array78/1
  Demux10/1 -> PV Array8/1
  Demux10/2 -> PV Array17/1
  Demux10/3 -> PV Array34/1
  Demux10/4 -> PV Array27/1
  Demux10/5 -> PV Array70/1
  Demux10/6 -> PV Array45/1
  Demux10/7 -> PV Array64/1
  Demux10/8 -> PV Array56/1
  Demux10/9 -> PV Array79/1
  In8/1 -> Demux10/1
  In7/1 -> Demux9/1
  In6/1 -> Demux8/1
  In5/1 -> Demux7/1
  In4/1 -> Demux6/1
  In3/1 -> Demux5/1
  In10/1 -> Demux4/1
  In2/1 -> Demux3/1
  connections:
  PV Array1/RConn2 -- Diode1/LConn1 -- PV Array2/RConn1 -- Diode2/RConn1 -- Diode11/RConn1 -- PV Array11/RConn1 -- PV Array10/RConn2 -- Diode10/LConn1 -- Diode28/RConn1 -- PV Array28/RConn1 -- PV Array19/RConn2 -- Diode19/LConn1 -- Diode20/LConn1 -- PV Array20/RConn2 -- PV Array21/RConn1 -- Diode21/RConn1 -- Diode48/RConn1 -- PV Array48/RConn1 -- PV Array37/RConn2 -- Diode37/LConn1 -- Diode38/LConn1 -- PV Array38/RConn2 -- PV Array39/RConn1 -- Diode39/RConn1 -- Diode47/LConn1 -- PV Array47/RConn2 -- PV Array57/RConn1 -- Diode57/RConn1 -- Diode50/RConn1 -- PV Array50/RConn1 -- PV Array49/RConn2 -- Diode49/LConn1 -- PV Array73/RConn1 -- Diode73/RConn1 -- Diode72/LConn1 -- PV Array72/RConn2
  Diode52/RConn1 -- PV Array52/RConn1 -- PV Array51/RConn2 -- Diode51/LConn1 -- Diode58/LConn1 -- PV Array58/RConn2 -- Diode60/RConn1 -- PV Array60/RConn1 -- Diode40/LConn1 -- PV Array40/RConn2 -- Diode41/RConn1 -- PV Array41/RConn1 -- Diode3/LConn1 -- PV Array3/RConn2 -- Diode4/RConn1 -- PV Array4/RConn1 -- Diode13/RConn1 -- PV Array13/RConn1 -- PV Array12/RConn2 -- Diode12/LConn1 -- Diode30/RConn1 -- PV Array30/RConn1 -- PV Array29/RConn2 -- Diode29/LConn1 -- Diode22/LConn1 -- PV Array22/RConn2 -- Diode23/RConn1 -- PV Array23/RConn1 -- Diode66/RConn1 -- PV Array66/RConn1 -- PV Array59/RConn2 -- Diode59/LConn1 -- Diode75/RConn1 -- PV Array75/RConn1 -- Diode74/LConn1 -- PV Array74/RConn2
  PV Array52/RConn2 -- Diode52/LConn1 -- PV Array60/RConn2 -- Diode60/LConn1 -- PV Array23/RConn2 -- Diode23/LConn1 -- PV Array4/RConn2 -- Diode4/LConn1 -- PV Array5/RConn1 -- Diode5/RConn1 -- PV Array13/RConn2 -- Diode13/LConn1 -- Diode14/RConn1 -- PV Array14/RConn1 -- PV Array30/RConn2 -- Diode30/LConn1 -- Diode31/RConn1 -- PV Array31/RConn1 -- PV Array24/RConn1 -- Diode24/RConn1 -- PV Array66/RConn2 -- Diode66/LConn1 -- Diode67/RConn1 -- PV Array67/RConn1 -- PV Array41/RConn2 -- Diode41/LConn1 -- PV Array42/RConn1 -- Diode42/RConn1 -- PV Array61/RConn1 -- Diode61/RConn1 -- Diode53/RConn1 -- PV Array53/RConn1 -- PV Array75/RConn2 -- Diode75/LConn1 -- PV Array76/RConn1 -- Diode76/RConn1
  Diode49/RConn1 -- PV Array49/RConn1 -- PV Array65/RConn2 -- Diode65/LConn1 -- Diode46/LConn1 -- PV Array46/RConn2 -- PV Array47/RConn1 -- Diode47/RConn1 -- Diode35/LConn1 -- PV Array35/RConn2 -- PV Array20/RConn1 -- Diode20/RConn1 -- Diode/LConn1 -- PV Array/RConn2 -- PV Array1/RConn1 -- Diode1/RConn1 -- Diode10/RConn1 -- PV Array10/RConn1 -- PV Array9/RConn2 -- Diode9/LConn1 -- Diode19/RConn1 -- PV Array19/RConn1 -- PV Array18/RConn2 -- Diode18/LConn1 -- Diode37/RConn1 -- PV Array37/RConn1 -- PV Array36/RConn2 -- Diode36/LConn1 -- Diode71/LConn1 -- PV Array71/RConn2 -- PV Array38/RConn1 -- Diode38/RConn1 -- PV Array72/RConn1 -- Diode72/RConn1 -- Diode80/LConn1 -- PV Array80/RConn2
  PV Array8/RConn2 -- PV Array34/RConn2 -- Diode34/LConn1 -- PV Array27/RConn2 -- Diode27/LConn1 -- PV Array70/RConn2 -- Diode70/LConn1 -- PV Array45/RConn2 -- Diode45/LConn1 -- PV Array64/RConn2 -- Diode64/LConn1 -- -/RConn1 -- PV Array79/RConn2 -- Diode79/LConn1 -- PV Array56/RConn2 -- Diode56/LConn1 -- PV Array17/RConn2 -- Diode17/LConn1 -- Diode8/LConn1
  Diode56/RConn1 -- PV Array56/RConn1 -- PV Array55/RConn2 -- Diode55/LConn1 -- Diode63/LConn1 -- PV Array63/RConn2 -- Diode64/RConn1 -- PV Array64/RConn1 -- Diode44/LConn1 -- PV Array44/RConn2 -- Diode45/RConn1 -- PV Array45/RConn1 -- Diode8/RConn1 -- PV Array8/RConn1 -- Diode7/LConn1 -- PV Array7/RConn2 -- Diode17/RConn1 -- PV Array17/RConn1 -- PV Array16/RConn2 -- Diode16/LConn1 -- Diode34/RConn1 -- PV Array34/RConn1 -- PV Array33/RConn2 -- Diode33/LConn1 -- Diode26/LConn1 -- PV Array26/RConn2 -- Diode27/RConn1 -- PV Array27/RConn1 -- Diode70/RConn1 -- PV Array70/RConn1 -- PV Array69/RConn2 -- Diode69/LConn1 -- Diode79/RConn1 -- PV Array79/RConn1 -- Diode78/LConn1 -- PV Array78/RConn2
  PV Array2/RConn2 -- Diode2/LConn1 -- PV Array3/RConn1 -- Diode3/RConn1 -- Diode12/RConn1 -- PV Array12/RConn1 -- PV Array11/RConn2 -- Diode11/LConn1 -- Diode29/RConn1 -- PV Array29/RConn1 -- PV Array28/RConn2 -- Diode28/LConn1 -- Diode21/LConn1 -- PV Array21/RConn2 -- PV Array22/RConn1 -- Diode22/RConn1 -- Diode59/RConn1 -- PV Array59/RConn1 -- PV Array48/RConn2 -- Diode48/LConn1 -- Diode39/LConn1 -- PV Array39/RConn2 -- PV Array40/RConn1 -- Diode40/RConn1 -- Diode57/LConn1 -- PV Array57/RConn2 -- PV Array58/RConn1 -- Diode58/RConn1 -- Diode51/RConn1 -- PV Array51/RConn1 -- PV Array50/RConn2 -- Diode50/LConn1 -- PV Array74/RConn1 -- Diode74/RConn1 -- Diode73/LConn1 -- PV Array73/RConn2
  PV Array78/RConn1 -- Diode78/RConn1 -- Diode77/LConn1 -- PV Array77/RConn2 -- Diode55/RConn1 -- PV Array55/RConn1 -- PV Array54/RConn2 -- Diode54/LConn1 -- PV Array63/RConn1 -- Diode63/RConn1 -- Diode62/LConn1 -- PV Array62/RConn2 -- PV Array44/RConn1 -- Diode44/RConn1 -- Diode43/LConn1 -- PV Array43/RConn2 -- Diode69/RConn1 -- PV Array69/RConn1 -- PV Array68/RConn2 -- Diode68/LConn1 -- PV Array26/RConn1 -- Diode26/RConn1 -- Diode25/LConn1 -- PV Array25/RConn2 -- Diode33/RConn1 -- PV Array33/RConn1 -- PV Array32/RConn2 -- Diode32/LConn1 -- Diode16/RConn1 -- PV Array16/RConn1 -- PV Array15/RConn2 -- Diode15/LConn1 -- Diode6/LConn1 -- PV Array6/RConn2 -- PV Array7/RConn1 -- Diode7/RConn1
  PV Array5/RConn2 -- Diode5/LConn1 -- PV Array6/RConn1 -- Diode6/RConn1 -- Diode15/RConn1 -- PV Array15/RConn1 -- PV Array14/RConn2 -- Diode14/LConn1 -- Diode32/RConn1 -- PV Array32/RConn1 -- PV Array31/RConn2 -- Diode31/LConn1 -- Diode24/LConn1 -- PV Array24/RConn2 -- PV Array25/RConn1 -- Diode25/RConn1 -- Diode68/RConn1 -- PV Array68/RConn1 -- PV Array67/RConn2 -- Diode67/LConn1 -- Diode42/LConn1 -- PV Array42/RConn2 -- PV Array43/RConn1 -- Diode43/RConn1 -- Diode61/LConn1 -- PV Array61/RConn2 -- PV Array62/RConn1 -- Diode62/RConn1 -- Diode54/RConn1 -- PV Array54/RConn1 -- PV Array53/RConn2 -- Diode53/LConn1 -- PV Array77/RConn1 -- Diode77/RConn1 -- Diode76/LConn1 -- PV Array76/RConn2
  PV Array18/RConn1 -- Diode18/RConn1 -- Diode35/RConn1 -- PV Array35/RConn1 -- Diode36/RConn1 -- PV Array36/RConn1 -- Diode71/RConn1 -- PV Array71/RConn1 -- Diode46/RConn1 -- PV Array46/RConn1 -- Diode65/RConn1 -- PV Array65/RConn1 -- PV Array80/RConn1 -- Diode80/RConn1 -- +/RConn1 -- Diode/RConn1 -- PV Array/RConn1 -- Diode9/RConn1 -- PV Array9/RConn1

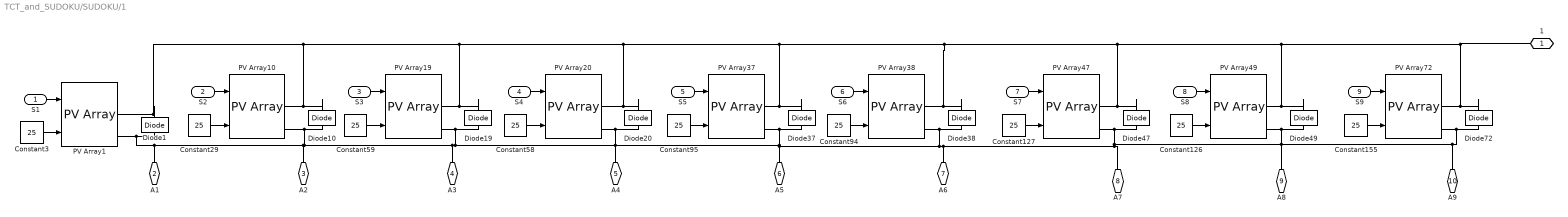
== system TCT_and_SUDOKU/SUDOKU/1 ==
  S1 : Inport
  S2 : Inport  Port=2
  S3 : Inport  Port=3
  S4 : Inport  Port=4
  S5 : Inport  Port=5
  S6 : Inport  Port=6
  S7 : Inport  Port=7
  S8 : Inport  Port=8
  S9 : Inport  Port=9
  Constant{3,29,58..59,94..95,126..127,155} (9 alike) : Constant  Value=25
  Diode{1,10,19..20,37..38,47,49,72} (9 alike) : spsDiodeLib/Diode  Ron=0.001  Lon=0  Vf=0.8  IC=0  UseSnubber=0  Rs=500  Cs=250e-9  Measurements=off
  PV Array{1,10,19..20,37..38,47,49,72} (9 alike) : spsPVArrayLib/PV Array  Npar=1  Nser=1  PlotType=array @ 1000 W/m2 & specified temperatures  S_vec="[ 1000  500  100 ]"  Temp_C_vec="[ 45 25  ]"  ModuleName=User-defined  PlotWhenSelected=off  Pm=79.2  Ncell=60  Voc=22  Isc=4.7  Vm=18  Im=4.4  beta_Voc_pc=-0.36099  alpha_Isc_pc=0.102  beta_Voc=-0.079418  alpha_Isc=0.004794  IL=4.7103  I0=1.7336e-10  nI=0.59447  Rsh=255.4401  Rs=0.29081  RobustModel=off  RobustCellTemperature=313.3991  BAL=on  Tc=1e-6  Tfilter=5e-5
  1 : PMIOPort  Side=Right
  A1 : PMIOPort  Port=2  Side=Right
  A2 : PMIOPort  Port=3  Side=Right
  A3 : PMIOPort  Port=4  Side=Right
  A4 : PMIOPort  Port=5  Side=Right
  A5 : PMIOPort  Port=6  Side=Right
  A6 : PMIOPort  Port=7  Side=Right
  A7 : PMIOPort  Port=8  Side=Right
  A8 : PMIOPort  Port=9  Side=Right
  A9 : PMIOPort  Port=10  Side=Right
  wires:
  S7/1 -> PV Array47/1
  Constant126/1 -> PV Array49/2
  S6/1 -> PV Array38/1
  S1/1 -> PV Array1/1
  Constant95/1 -> PV Array37/2
  S5/1 -> PV Array37/1
  Constant127/1 -> PV Array47/2
  Constant94/1 -> PV Array38/2
  S8/1 -> PV Array49/1
  S4/1 -> PV Array20/1
  Constant155/1 -> PV Array72/2
  Constant29/1 -> PV Array10/2
  Constant58/1 -> PV Array20/2
  Constant59/1 -> PV Array19/2
  S9/1 -> PV Array72/1
  Constant3/1 -> PV Array1/2
  S3/1 -> PV Array19/1
  S2/1 -> PV Array10/1
  connections:
  1/RConn1 -- PV Array49/RConn1 -- Diode49/RConn1 -- PV Array47/RConn1 -- Diode47/RConn1 -- PV Array38/RConn1 -- Diode38/RConn1 -- PV Array1/RConn1 -- Diode1/RConn1 -- PV Array10/RConn1 -- Diode10/RConn1 -- PV Array19/RConn1 -- Diode19/RConn1 -- PV Array20/RConn1 -- Diode20/RConn1 -- PV Array37/RConn1 -- Diode37/RConn1 -- PV Array72/RConn1 -- Diode72/RConn1
  PV Array38/RConn2 -- Diode38/LConn1 -- A5/RConn1 -- PV Array20/RConn2 -- Diode20/LConn1 -- A4/RConn1 -- PV Array19/RConn2 -- Diode19/LConn1 -- A3/RConn1 -- Diode10/LConn1 -- PV Array10/RConn2 -- A2/RConn1 -- A1/RConn1 -- Diode1/LConn1 -- PV Array1/RConn2 -- PV Array37/RConn2 -- Diode37/LConn1 -- A7/RConn1 -- PV Array49/RConn2 -- Diode49/LConn1 -- A9/RConn1 -- PV Array72/RConn2 -- Diode72/LConn1 -- A8/RConn1 -- PV Array47/RConn2 -- Diode47/LConn1 -- A6/RConn1

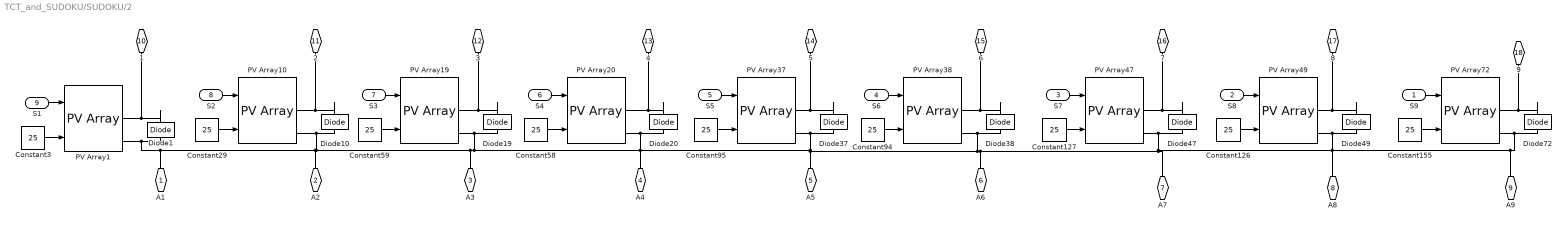
== system TCT_and_SUDOKU/SUDOKU/2 ==
  S9 : Inport
  S8 : Inport  Port=2
  S7 : Inport  Port=3
  S6 : Inport  Port=4
  S5 : Inport  Port=5
  S4 : Inport  Port=6
  S3 : Inport  Port=7
  S2 : Inport  Port=8
  S1 : Inport  Port=9
  Constant{3,29,58..59,94..95,126..127,155} (9 alike) : Constant  Value=25
  Diode{1,10,19..20,37..38,47,49,72} (9 alike) : spsDiodeLib/Diode  Ron=0.001  Lon=0  Vf=0.8  IC=0  UseSnubber=0  Rs=500  Cs=250e-9  Measurements=off
  PV Array{1,10,19..20,37..38,47,49,72} (9 alike) : spsPVArrayLib/PV Array  Npar=1  Nser=1  PlotType=array @ 1000 W/m2 & specified temperatures  S_vec="[ 1000  500  100 ]"  Temp_C_vec="[ 45 25  ]"  ModuleName=User-defined  PlotWhenSelected=off  Pm=79.2  Ncell=60  Voc=22  Isc=4.7  Vm=18  Im=4.4  beta_Voc_pc=-0.36099  alpha_Isc_pc=0.102  beta_Voc=-0.079418  alpha_Isc=0.004794  IL=4.7103  I0=1.7336e-10  nI=0.59447  Rsh=255.4401  Rs=0.29081  RobustModel=off  RobustCellTemperature=313.3991  BAL=on  Tc=1e-6  Tfilter=5e-5
  A1 : PMIOPort  Side=Left
  A2 : PMIOPort  Port=2  Side=Left
  A3 : PMIOPort  Port=3  Side=Left
  A4 : PMIOPort  Port=4  Side=Left
  A5 : PMIOPort  Port=5  Side=Left
  A6 : PMIOPort  Port=6  Side=Left
  A7 : PMIOPort  Port=7  Side=Left
  A8 : PMIOPort  Port=8  Side=Left
  A9 : PMIOPort  Port=9  Side=Left
  1 : PMIOPort  Port=10  Side=Right
  2 : PMIOPort  Port=11  Side=Right
  3 : PMIOPort  Port=12  Side=Right
  4 : PMIOPort  Port=13  Side=Right
  5 : PMIOPort  Port=14  Side=Right
  6 : PMIOPort  Port=15  Side=Right
  7 : PMIOPort  Port=16  Side=Right
  8 : PMIOPort  Port=17  Side=Right
  9 : PMIOPort  Port=18  Side=Right
  wires:
  S2/1 -> PV Array10/1
  S3/1 -> PV Array19/1
  Constant3/1 -> PV Array1/2
  S9/1 -> PV Array72/1
  Constant59/1 -> PV Array19/2
  Constant58/1 -> PV Array20/2
  Constant29/1 -> PV Array10/2
  Constant155/1 -> PV Array72/2
  S4/1 -> PV Array20/1
  S8/1 -> PV Array49/1
  Constant94/1 -> PV Array38/2
  Constant127/1 -> PV Array47/2
  S5/1 -> PV Array37/1
  Constant95/1 -> PV Array37/2
  S1/1 -> PV Array1/1
  S6/1 -> PV Array38/1
  Constant126/1 -> PV Array49/2
  S7/1 -> PV Array47/1
  connections:
  Diode10/RConn1 -- 2/RConn1 -- PV Array10/RConn1
  Diode20/RConn1 -- 4/RConn1 -- PV Array20/RConn1
  Diode19/RConn1 -- 3/RConn1 -- PV Array19/RConn1
  A6/RConn1 -- Diode47/LConn1 -- PV Array47/RConn2 -- A8/RConn1 -- Diode72/LConn1 -- PV Array72/RConn2 -- A9/RConn1 -- Diode49/LConn1 -- PV Array49/RConn2 -- A7/RConn1 -- Diode37/LConn1 -- PV Array37/RConn2 -- PV Array1/RConn2 -- Diode1/LConn1 -- A1/RConn1 -- A2/RConn1 -- PV Array10/RConn2 -- Diode10/LConn1 -- A3/RConn1 -- Diode19/LConn1 -- PV Array19/RConn2 -- A4/RConn1 -- Diode20/LConn1 -- PV Array20/RConn2 -- A5/RConn1 -- Diode38/LConn1 -- PV Array38/RConn2
  Diode47/RConn1 -- 7/RConn1 -- PV Array47/RConn1
  Diode49/RConn1 -- PV Array49/RConn1 -- 8/RConn1
  Diode1/RConn1 -- 1/RConn1 -- PV Array1/RConn1
  Diode72/RConn1 -- 9/RConn1 -- PV Array72/RConn1
  Diode37/RConn1 -- PV Array37/RConn1 -- 5/RConn1
  Diode38/RConn1 -- 6/RConn1 -- PV Array38/RConn1

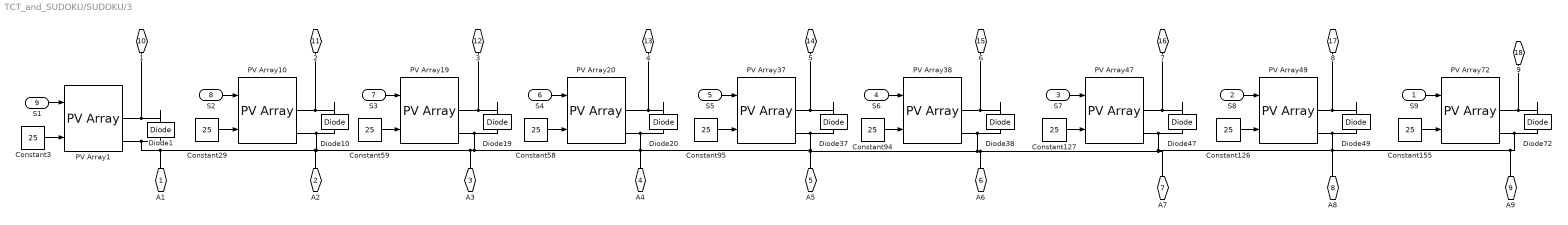
== system TCT_and_SUDOKU/SUDOKU/3 ==
  S9 : Inport
  S8 : Inport  Port=2
  S7 : Inport  Port=3
  S6 : Inport  Port=4
  S5 : Inport  Port=5
  S4 : Inport  Port=6
  S3 : Inport  Port=7
  S2 : Inport  Port=8
  S1 : Inport  Port=9
  Constant{3,29,58..59,94..95,126..127,155} (9 alike) : Constant  Value=25
  Diode{1,10,19..20,37..38,47,49,72} (9 alike) : spsDiodeLib/Diode  Ron=0.001  Lon=0  Vf=0.8  IC=0  UseSnubber=0  Rs=500  Cs=250e-9  Measurements=off
  PV Array{1,10,19..20,37..38,47,49,72} (9 alike) : spsPVArrayLib/PV Array  Npar=1  Nser=1  PlotType=array @ 1000 W/m2 & specified temperatures  S_vec="[ 1000  500  100 ]"  Temp_C_vec="[ 45 25  ]"  ModuleName=User-defined  PlotWhenSelected=off  Pm=79.2  Ncell=60  Voc=22  Isc=4.7  Vm=18  Im=4.4  beta_Voc_pc=-0.36099  alpha_Isc_pc=0.102  beta_Voc=-0.079418  alpha_Isc=0.004794  IL=4.7103  I0=1.7336e-10  nI=0.59447  Rsh=255.4401  Rs=0.29081  RobustModel=off  RobustCellTemperature=313.3991  BAL=on  Tc=1e-6  Tfilter=5e-5
  A1 : PMIOPort  Side=Left
  A2 : PMIOPort  Port=2  Side=Left
  A3 : PMIOPort  Port=3  Side=Left
  A4 : PMIOPort  Port=4  Side=Left
  A5 : PMIOPort  Port=5  Side=Left
  A6 : PMIOPort  Port=6  Side=Left
  A7 : PMIOPort  Port=7  Side=Left
  A8 : PMIOPort  Port=8  Side=Left
  A9 : PMIOPort  Port=9  Side=Left
  1 : PMIOPort  Port=10  Side=Right
  2 : PMIOPort  Port=11  Side=Right
  3 : PMIOPort  Port=12  Side=Right
  4 : PMIOPort  Port=13  Side=Right
  5 : PMIOPort  Port=14  Side=Right
  6 : PMIOPort  Port=15  Side=Right
  7 : PMIOPort  Port=16  Side=Right
  8 : PMIOPort  Port=17  Side=Right
  9 : PMIOPort  Port=18  Side=Right
  wires:
  S7/1 -> PV Array47/1
  Constant126/1 -> PV Array49/2
  S6/1 -> PV Array38/1
  S1/1 -> PV Array1/1
  Constant95/1 -> PV Array37/2
  S5/1 -> PV Array37/1
  Constant127/1 -> PV Array47/2
  Constant94/1 -> PV Array38/2
  S8/1 -> PV Array49/1
  S4/1 -> PV Array20/1
  Constant155/1 -> PV Array72/2
  Constant29/1 -> PV Array10/2
  Constant58/1 -> PV Array20/2
  Constant59/1 -> PV Array19/2
  S9/1 -> PV Array72/1
  Constant3/1 -> PV Array1/2
  S3/1 -> PV Array19/1
  S2/1 -> PV Array10/1
  connections:
  PV Array38/RConn1 -- 6/RConn1 -- Diode38/RConn1
  5/RConn1 -- PV Array37/RConn1 -- Diode37/RConn1
  PV Array72/RConn1 -- 9/RConn1 -- Diode72/RConn1
  PV Array1/RConn1 -- 1/RConn1 -- Diode1/RConn1
  8/RConn1 -- PV Array49/RConn1 -- Diode49/RConn1
  PV Array47/RConn1 -- 7/RConn1 -- Diode47/RConn1
  PV Array38/RConn2 -- Diode38/LConn1 -- A5/RConn1 -- PV Array20/RConn2 -- Diode20/LConn1 -- A4/RConn1 -- PV Array19/RConn2 -- Diode19/LConn1 -- A3/RConn1 -- Diode10/LConn1 -- PV Array10/RConn2 -- A2/RConn1 -- A1/RConn1 -- Diode1/LConn1 -- PV Array1/RConn2 -- PV Array37/RConn2 -- Diode37/LConn1 -- A7/RConn1 -- PV Array49/RConn2 -- Diode49/LConn1 -- A9/RConn1 -- PV Array72/RConn2 -- Diode72/LConn1 -- A8/RConn1 -- PV Array47/RConn2 -- Diode47/LConn1 -- A6/RConn1
  PV Array19/RConn1 -- 3/RConn1 -- Diode19/RConn1
  PV Array20/RConn1 -- 4/RConn1 -- Diode20/RConn1
  PV Array10/RConn1 -- 2/RConn1 -- Diode10/RConn1

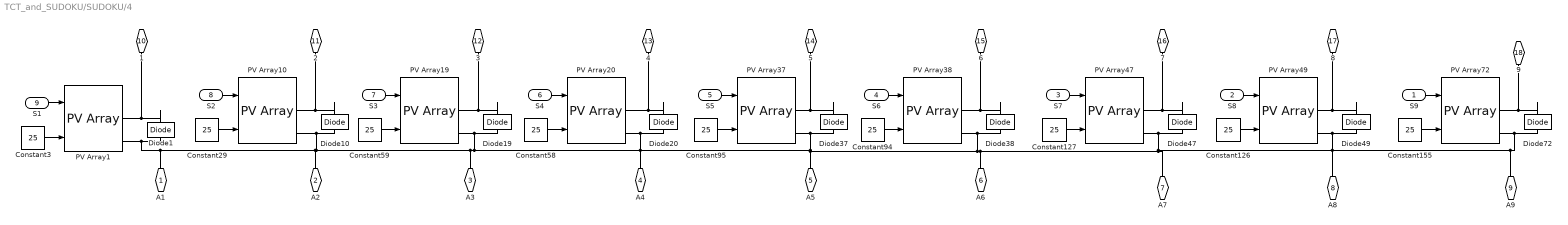
== system TCT_and_SUDOKU/SUDOKU/4 ==
  S9 : Inport
  S8 : Inport  Port=2
  S7 : Inport  Port=3
  S6 : Inport  Port=4
  S5 : Inport  Port=5
  S4 : Inport  Port=6
  S3 : Inport  Port=7
  S2 : Inport  Port=8
  S1 : Inport  Port=9
  Constant{3,29,58..59,94..95,126..127,155} (9 alike) : Constant  Value=25
  Diode{1,10,19..20,37..38,47,49,72} (9 alike) : spsDiodeLib/Diode  Ron=0.001  Lon=0  Vf=0.8  IC=0  UseSnubber=0  Rs=500  Cs=250e-9  Measurements=off
  PV Array{1,10,19..20,37..38,47,49,72} (9 alike) : spsPVArrayLib/PV Array  Npar=1  Nser=1  PlotType=array @ 1000 W/m2 & specified temperatures  S_vec="[ 1000  500  100 ]"  Temp_C_vec="[ 45 25  ]"  ModuleName=User-defined  PlotWhenSelected=off  Pm=79.2  Ncell=60  Voc=22  Isc=4.7  Vm=18  Im=4.4  beta_Voc_pc=-0.36099  alpha_Isc_pc=0.102  beta_Voc=-0.079418  alpha_Isc=0.004794  IL=4.7103  I0=1.7336e-10  nI=0.59447  Rsh=255.4401  Rs=0.29081  RobustModel=off  RobustCellTemperature=313.3991  BAL=on  Tc=1e-6  Tfilter=5e-5
  A1 : PMIOPort  Side=Left
  A2 : PMIOPort  Port=2  Side=Left
  A3 : PMIOPort  Port=3  Side=Left
  A4 : PMIOPort  Port=4  Side=Left
  A5 : PMIOPort  Port=5  Side=Left
  A6 : PMIOPort  Port=6  Side=Left
  A7 : PMIOPort  Port=7  Side=Left
  A8 : PMIOPort  Port=8  Side=Left
  A9 : PMIOPort  Port=9  Side=Left
  1 : PMIOPort  Port=10  Side=Right
  2 : PMIOPort  Port=11  Side=Right
  3 : PMIOPort  Port=12  Side=Right
  4 : PMIOPort  Port=13  Side=Right
  5 : PMIOPort  Port=14  Side=Right
  6 : PMIOPort  Port=15  Side=Right
  7 : PMIOPort  Port=16  Side=Right
  8 : PMIOPort  Port=17  Side=Right
  9 : PMIOPort  Port=18  Side=Right
  wires:
  S2/1 -> PV Array10/1
  S3/1 -> PV Array19/1
  Constant3/1 -> PV Array1/2
  S9/1 -> PV Array72/1
  Constant59/1 -> PV Array19/2
  Constant58/1 -> PV Array20/2
  Constant29/1 -> PV Array10/2
  Constant155/1 -> PV Array72/2
  S4/1 -> PV Array20/1
  S8/1 -> PV Array49/1
  Constant94/1 -> PV Array38/2
  Constant127/1 -> PV Array47/2
  S5/1 -> PV Array37/1
  Constant95/1 -> PV Array37/2
  S1/1 -> PV Array1/1
  S6/1 -> PV Array38/1
  Constant126/1 -> PV Array49/2
  S7/1 -> PV Array47/1
  connections:
  Diode10/RConn1 -- 2/RConn1 -- PV Array10/RConn1
  Diode20/RConn1 -- 4/RConn1 -- PV Array20/RConn1
  Diode19/RConn1 -- 3/RConn1 -- PV Array19/RConn1
  A6/RConn1 -- Diode47/LConn1 -- PV Array47/RConn2 -- A8/RConn1 -- Diode72/LConn1 -- PV Array72/RConn2 -- A9/RConn1 -- Diode49/LConn1 -- PV Array49/RConn2 -- A7/RConn1 -- Diode37/LConn1 -- PV Array37/RConn2 -- PV Array1/RConn2 -- Diode1/LConn1 -- A1/RConn1 -- A2/RConn1 -- PV Array10/RConn2 -- Diode10/LConn1 -- A3/RConn1 -- Diode19/LConn1 -- PV Array19/RConn2 -- A4/RConn1 -- Diode20/LConn1 -- PV Array20/RConn2 -- A5/RConn1 -- Diode38/LConn1 -- PV Array38/RConn2
  Diode47/RConn1 -- 7/RConn1 -- PV Array47/RConn1
  Diode49/RConn1 -- PV Array49/RConn1 -- 8/RConn1
  Diode1/RConn1 -- 1/RConn1 -- PV Array1/RConn1
  Diode72/RConn1 -- 9/RConn1 -- PV Array72/RConn1
  Diode37/RConn1 -- PV Array37/RConn1 -- 5/RConn1
  Diode38/RConn1 -- 6/RConn1 -- PV Array38/RConn1

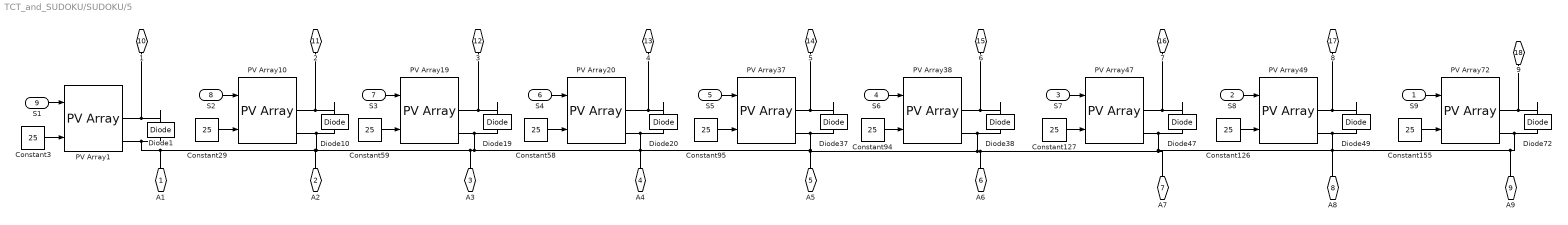
== system TCT_and_SUDOKU/SUDOKU/5 ==
  S9 : Inport
  S8 : Inport  Port=2
  S7 : Inport  Port=3
  S6 : Inport  Port=4
  S5 : Inport  Port=5
  S4 : Inport  Port=6
  S3 : Inport  Port=7
  S2 : Inport  Port=8
  S1 : Inport  Port=9
  Constant{3,29,58..59,94..95,126..127,155} (9 alike) : Constant  Value=25
  Diode{1,10,19..20,37..38,47,49,72} (9 alike) : spsDiodeLib/Diode  Ron=0.001  Lon=0  Vf=0.8  IC=0  UseSnubber=0  Rs=500  Cs=250e-9  Measurements=off
  PV Array{1,10,19..20,37..38,47,49,72} (9 alike) : spsPVArrayLib/PV Array  Npar=1  Nser=1  PlotType=array @ 1000 W/m2 & specified temperatures  S_vec="[ 1000  500  100 ]"  Temp_C_vec="[ 45 25  ]"  ModuleName=User-defined  PlotWhenSelected=off  Pm=79.2  Ncell=60  Voc=22  Isc=4.7  Vm=18  Im=4.4  beta_Voc_pc=-0.36099  alpha_Isc_pc=0.102  beta_Voc=-0.079418  alpha_Isc=0.004794  IL=4.7103  I0=1.7336e-10  nI=0.59447  Rsh=255.4401  Rs=0.29081  RobustModel=off  RobustCellTemperature=313.3991  BAL=on  Tc=1e-6  Tfilter=5e-5
  A1 : PMIOPort  Side=Left
  A2 : PMIOPort  Port=2  Side=Left
  A3 : PMIOPort  Port=3  Side=Left
  A4 : PMIOPort  Port=4  Side=Left
  A5 : PMIOPort  Port=5  Side=Left
  A6 : PMIOPort  Port=6  Side=Left
  A7 : PMIOPort  Port=7  Side=Left
  A8 : PMIOPort  Port=8  Side=Left
  A9 : PMIOPort  Port=9  Side=Left
  1 : PMIOPort  Port=10  Side=Right
  2 : PMIOPort  Port=11  Side=Right
  3 : PMIOPort  Port=12  Side=Right
  4 : PMIOPort  Port=13  Side=Right
  5 : PMIOPort  Port=14  Side=Right
  6 : PMIOPort  Port=15  Side=Right
  7 : PMIOPort  Port=16  Side=Right
  8 : PMIOPort  Port=17  Side=Right
  9 : PMIOPort  Port=18  Side=Right
  wires:
  S7/1 -> PV Array47/1
  Constant126/1 -> PV Array49/2
  S6/1 -> PV Array38/1
  S1/1 -> PV Array1/1
  Constant95/1 -> PV Array37/2
  S5/1 -> PV Array37/1
  Constant127/1 -> PV Array47/2
  Constant94/1 -> PV Array38/2
  S8/1 -> PV Array49/1
  S4/1 -> PV Array20/1
  Constant155/1 -> PV Array72/2
  Constant29/1 -> PV Array10/2
  Constant58/1 -> PV Array20/2
  Constant59/1 -> PV Array19/2
  S9/1 -> PV Array72/1
  Constant3/1 -> PV Array1/2
  S3/1 -> PV Array19/1
  S2/1 -> PV Array10/1
  connections:
  PV Array38/RConn1 -- 6/RConn1 -- Diode38/RConn1
  5/RConn1 -- PV Array37/RConn1 -- Diode37/RConn1
  PV Array72/RConn1 -- 9/RConn1 -- Diode72/RConn1
  PV Array1/RConn1 -- 1/RConn1 -- Diode1/RConn1
  8/RConn1 -- PV Array49/RConn1 -- Diode49/RConn1
  PV Array47/RConn1 -- 7/RConn1 -- Diode47/RConn1
  PV Array38/RConn2 -- Diode38/LConn1 -- A5/RConn1 -- PV Array20/RConn2 -- Diode20/LConn1 -- A4/RConn1 -- PV Array19/RConn2 -- Diode19/LConn1 -- A3/RConn1 -- Diode10/LConn1 -- PV Array10/RConn2 -- A2/RConn1 -- A1/RConn1 -- Diode1/LConn1 -- PV Array1/RConn2 -- PV Array37/RConn2 -- Diode37/LConn1 -- A7/RConn1 -- PV Array49/RConn2 -- Diode49/LConn1 -- A9/RConn1 -- PV Array72/RConn2 -- Diode72/LConn1 -- A8/RConn1 -- PV Array47/RConn2 -- Diode47/LConn1 -- A6/RConn1
  PV Array19/RConn1 -- 3/RConn1 -- Diode19/RConn1
  PV Array20/RConn1 -- 4/RConn1 -- Diode20/RConn1
  PV Array10/RConn1 -- 2/RConn1 -- Diode10/RConn1
